simulink model "FOC_fieldWeakening"  (R2023b)
settings: Solver=FixedStepDiscrete  StartTime=0.0  StopTime=3  RelTol=1e-3  EnableMultiTasking=on
InitFcn:
  | mcb_pmsm_fwc_qep_f28379d_data;
model workspace (MAT data in the model file):
  encoderResolution = 2000
  hallOffset = '0.5'
  indexOffset = 850
  polePairs = '4'
values from neighbouring files (symbols this model uses):
  A = 42    [TestigAdder.m]
  dataType = 'single'    [FOC_Param.m]    (also in FOC_simulationParameters.m; mcb_pmsm_fwc_qep_f28379d_data.m; open_loop_control_script.m = fixdt(1,32,17))
  inverter = mcb_updateInverterParameters(pmsm,inverter,target)    [FOC_Param.m]    (also in FOC_simulationParameters.m = mcb_SetInverterParameters('BoostXL-DRV8301'); mcb_pmsm_fwc_qep_f28379d_data.m = mcb_SetInverterParameters('BoostXL-DRV8305'))
  maxMotorCurrent = pmsm.I_rated    [mcb_pmsm_fwc_qep_f28379d_data.m]
  PI_params = mcb_SetControllerParameters(pmsm,inverter,PU_System,T_pwm,Ts,Ts_speed)    [FOC_Param.m]    (also in FOC_simulationParameters.m = mcb_SetControllerParameters(pmsm,inverter,PU_System,T_pwm,2*; mcb_pmsm_fwc_qep_f28379d_data.m = mcb_SetControllerParameters(pmsm,inverter,PU_System,T_pwm,Ts)
  pmsm = mcb_SetPMSMMotorParameters('Teknic2310P')    [FOC_Param.m]    (also in FOC_simulationParameters.m; mcb_pmsm_fwc_qep_f28379d_data.m)
  PU_System = mcb_SetPUSystem(pmsm,inverter)    [FOC_Param.m]    (also in FOC_simulationParameters.m; mcb_pmsm_fwc_qep_f28379d_data.m)
  target = mcb_SetProcessorDetails('F28379D',PWM_frequency)    [FOC_Param.m]    (also in FOC_simulationParameters.m; mcb_pmsm_fwc_qep_f28379d_data.m)
  Ts = T_pwm    (= 5e-05)    [FOC_Param.m]    (also in FOC_simulationParameters.m; mcb_pmsm_fwc_qep_f28379d_data.m; open_loop_control_script.m = T_pwm)
  Ts_speed = 10*Ts    (= 0.0005)    [FOC_Param.m]    (also in FOC_simulationParameters.m = 0.001; mcb_pmsm_fwc_qep_f28379d_data.m = 0.0015)
undefined symbols (not defined in the file or in its folder): Down, GPTRIP1SEL, GPTRIP2SEL, TZ1, TZ2, Up
libraries: simulink x17, mcbcontrolslib x11, c280xlib x10, c2802xlib x7, svdutilitieslib x7, slpidlib x4, c2837xDlib x3, mcbpositiondecoderlib x3, mcbpmsmnonlinearlib x2, svdschedulerlib x2
(part 2 of 3)

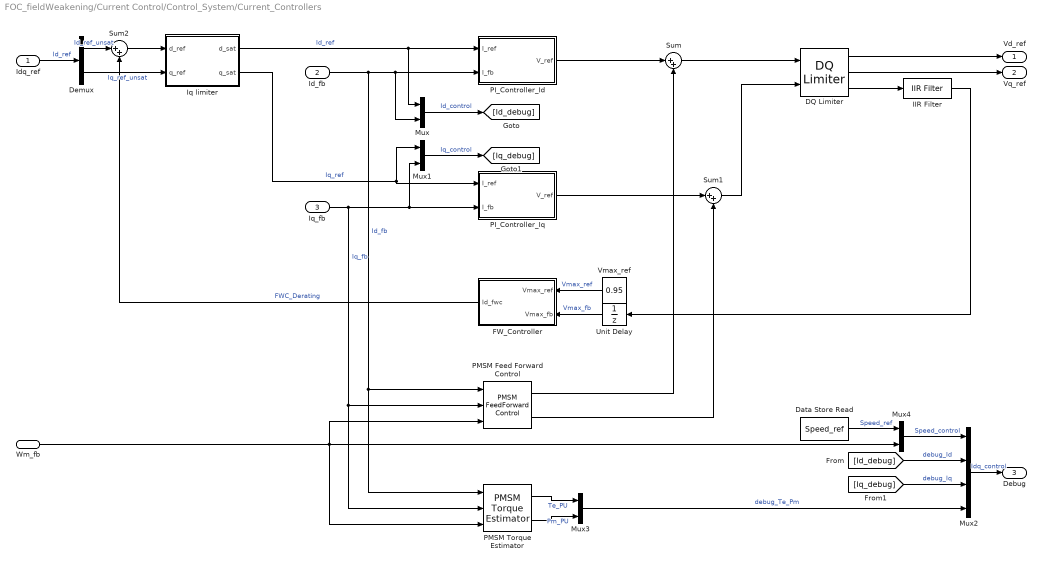
== system FOC_fieldWeakening/Current Control/Control_System/Current_Controllers ==
  Idq_ref : Inport
  Id_fb : Inport  Port=2
  Iq_fb : Inport  Port=3
  Wm_fb : Inport  Port=4
  DQ Limiter : mcbcontrolslib/DQ Limiter  satMethodInputType=Specify via dialog  satMethodSelected=D-Q equivalence  satLimitInputType=Specify via dialog  Vmax=0.95
  Data Store Read : DataStoreRead  DataStoreName=Speed_ref  IndexOptions=Index vector (dialog)  Indices=1  OutputSizes=1
  Demux : Demux  Outputs=2
  FW_Controller : Subsystem
  IIR Filter : mcbcontrolslib/IIR Filter  VariantControl=Low Pass Filter  VariantSelect=Low-pass  Filter_constant=0.01  advancedSettings=off  Ts=50e-6  cutOff_freq=32.1525
  Iq limiter : Subsystem
  Mux{,1,3..4} (4 alike) : Mux  Inputs=2
  Mux2 : Mux
  PI_Controller_Id : Subsystem
  PI_Controller_Iq : Subsystem
  PMSM Feed Forward Control : mcbpmsmnonlinearlib/PMSM FeedForward Control  polePairs=pmsm.p  nonLinearityChoice=Linear model with lumped parameters  Ld=pmsm.Ld  Lq=pmsm.Lq  FluxPM=pmsm.FluxPM  idVec=[-40, -20, 0, 20]  iqVec=[-40, -20, 0, 20, 40]  LdTable=0.2e-3 * ones(4, 5)  LqTable=0.2e-3 * ones(4, 5)  FluxPMTable=6.4e-3 * ones(4, 5)  FluxDTable=[-1.6,-1.6,-1.6,-1.6,-1.6;2.4,2.4,2.4,2.4,2.4;6.4,6.4,6.4,6.4,6.4;10.4,10.4,10.4,10.4,10.4]*1e-3  FluxQTable=[-8,-4,0,4,8;-8,-4,0,4,8;-8,-4,0,4,8;-8,-4,0,4,8]*1e-3  Vsat_input_select=Specify via dialog  v_sat=0.05*PU_System.V_base  Units=Per-Unit (PU)  V_base=PU_System.V_base  I_base=PU_System.I_base  N_base=PU_System.N_base  scaledTables=on
  PMSM Torque Estimator : mcbpmsmnonlinearlib/PMSM Torque Estimator  polePairs=pmsm.p  nonLinearityChoice=Linear model with lumped parameters  Ld=pmsm.Ld  Lq=pmsm.Lq  FluxPM=pmsm.FluxPM  idVec=[-40, -20, 0, 20]  iqVec=[-40, -20, 0, 20, 40]  LdTable=0.2e-3 * ones(4, 5)  LqTable=0.2e-3 * ones(4, 5)  FluxPMTable=6.4e-3 * ones(4, 5)  FluxDTable=[-1.6,-1.6,-1.6,-1.6,-1.6;2.4,2.4,2.4,2.4,2.4;6.4,6.4,6.4,6.4,6.4;10.4,10.4,10.4,10.4,10.4]*1e-3  FluxQTable=[-8,-4,0,4,8;-8,-4,0,4,8;-8,-4,0,4,8;-8,-4,0,4,8]*1e-3  Units=Per-Unit (PU)  V_base=PU_System.V_base  I_base=PU_System.I_base  N_base=PU_System.N_base  T_base=0.82227  P_base=445.3845  scaledTables=on
  Sum : Sum  Inputs=|++
  Sum1 : Sum  Inputs=|++
  Sum2 : Sum  Inputs=|++
  Unit Delay : UnitDelay  SampleTime=-1  HasFrameUpgradeWarning=on
  Vmax_ref : Constant  Value=0.95  OutDataTypeStr=dataType  SampleTime=-1
  Vd_ref : Outport  VectorParamsAs1DForOutWhenUnconnected=off
  Vq_ref : Outport  Port=2  VectorParamsAs1DForOutWhenUnconnected=off
  Debug : Outport  Port=3  VectorParamsAs1DForOutWhenUnconnected=off
  wires:
  Mux/1 -> [Id_debug]  "Id_control"
  Id_fb/1 -> PMSM Torque Estimator/1, PMSM Feed Forward Control/1, Mux/2, PI_Controller_Id/2(I_fb)  "Id_fb"
  Mux1/1 -> [Iq_debug]  "Iq_control"
  DQ Limiter/1 -> Vd_ref/1
  DQ Limiter/2 -> Vq_ref/1
  PI_Controller_Id/1(V_ref) -> Sum/1
  PMSM Torque Estimator/1 -> Mux3/1  "Te_PU"
  FW_Controller/1(Id_fwc) -> Sum2/2  "FWC_Derating"
  Vmax_ref/1 -> FW_Controller/1(Vmax_ref)  "Vmax_ref"
  Iq_fb/1 -> PMSM Torque Estimator/2, PMSM Feed Forward Control/2, PI_Controller_Iq/2(I_fb), Mux1/2  "Iq_fb"
  PI_Controller_Iq/1(V_ref) -> Sum1/1
  Sum1/1 -> DQ Limiter/2
  Sum/1 -> DQ Limiter/1
  Iq limiter/2(q_sat) -> PI_Controller_Iq/1(I_ref), Mux1/1  "Iq_ref"
  Unit Delay/1 -> FW_Controller/2(Vmax_fb)  "Vmax_fb"
  IIR Filter/1 -> Unit Delay/1
  DQ Limiter/3 -> IIR Filter/1
  PMSM Feed Forward Control/1 -> Sum/2
  PMSM Feed Forward Control/2 -> Sum1/2
  Idq_ref/1 -> Demux/1  "Id_ref"
  Mux2/1 -> Debug/1  "Idq_control"
  [Id_debug] -> Mux2/2  "debug_Id"
  [Iq_debug] -> Mux2/3  "debug_Iq"
  PMSM Torque Estimator/2 -> Mux3/2  "Pm_PU"
  Mux3/1 -> Mux2/4  "debug_Te_Pm"
  Mux4/1 -> Mux2/1  "Speed_control"
  Wm_fb/1 -> PMSM Torque Estimator/3, PMSM Feed Forward Control/3, Mux4/2
  Data Store Read/1 -> Mux4/1  "Speed_ref"
  Iq limiter/1(d_sat) -> PI_Controller_Id/1(I_ref), Mux/1  "Id_ref"
  Sum2/1 -> Iq limiter/1(d_ref)
  Demux/1 -> Sum2/1  "Id_ref_unsat"
  Demux/2 -> Iq limiter/2(q_ref)  "Iq_ref_unsat"

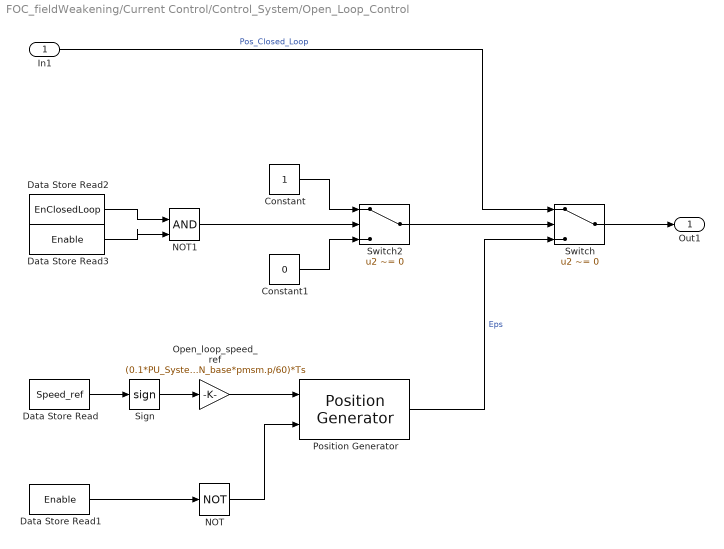
== system FOC_fieldWeakening/Current Control/Control_System/Open_Loop_Control ==
  In1 : Inport
  Constant : Constant  OutDataTypeStr=uint16
  Constant1 : Constant  Value=0  OutDataTypeStr=uint16
  Data Store Read : DataStoreRead  DataStoreName=Speed_ref  IndexOptions=Index vector (dialog)  Indices=1  OutputSizes=1
  Data Store Read1 : DataStoreRead  DataStoreName=Enable  IndexOptions=Index vector (dialog)  Indices=1  OutputSizes=1
  Data Store Read2 : DataStoreRead  DataStoreName=EnClosedLoop  IndexOptions=Index vector (dialog)  Indices=1  OutputSizes=1
  Data Store Read3 : DataStoreRead  DataStoreName=Enable  IndexOptions=Index vector (dialog)  Indices=1  OutputSizes=1
  NOT : Logic  Operator=NOT  IconShape=distinctive  AllPortsSameDT=off  OutDataTypeStr=boolean
  NOT1 : Logic  IconShape=distinctive  AllPortsSameDT=off  OutDataTypeStr=boolean
  Open_loop_speed_ref : Gain  Gain=(0.1*PU_System.N_base*pmsm.p/60)*Ts  ParamDataTypeStr=dataType  OutDataTypeStr=dataType  RndMeth=Simplest
  Position Generator : mcbcontrolslib/Position Generator  AngleOutput=Per-unit  ExternalReset=active high resets to zero  Offset=0
  Sign : Signum
  Switch : Switch  Criteria=u2 ~= 0  Threshold=0.1  SaturateOnIntegerOverflow=off  InputSameDT=off
  Switch2 : Switch  Criteria=u2 ~= 0  SaturateOnIntegerOverflow=off  InputSameDT=off
  Out1 : Outport
  wires:
  Constant1/1 -> Switch2/3
  Constant/1 -> Switch2/1
  In1/1 -> Switch/1  "Pos_Closed_Loop"
  Switch/1 -> Out1/1
  Open_loop_speed_ref/1 -> Position Generator/1
  Switch2/1 -> Switch/2
  Data Store Read/1 -> Sign/1
  Position Generator/1 -> Switch/3  "Eps"
  Data Store Read1/1 -> NOT/1
  NOT/1 -> Position Generator/2
  Data Store Read2/1 -> NOT1/1
  Data Store Read3/1 -> NOT1/2
  NOT1/1 -> Switch2/2
  Sign/1 -> Open_loop_speed_ref/1

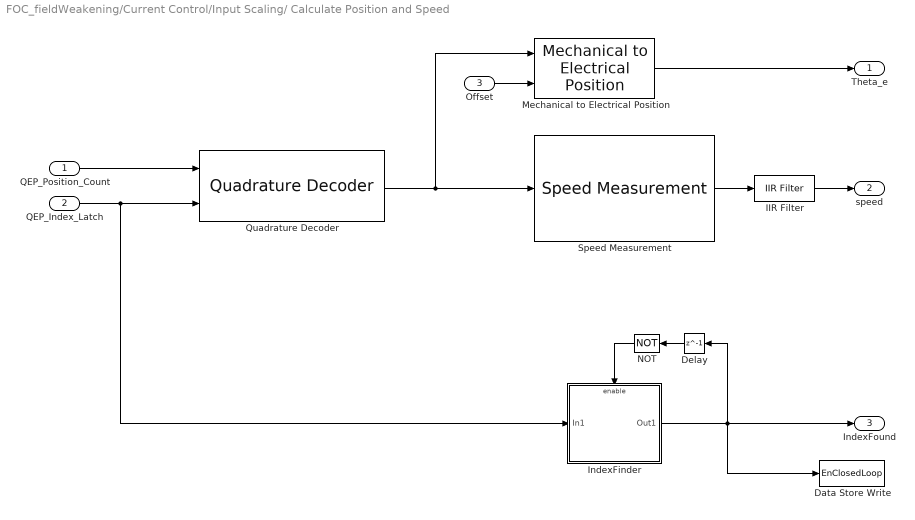
== system FOC_fieldWeakening/Current Control/Input Scaling/ Calculate Position and Speed ==
  QEP_Position_Count : Inport
  QEP_Index_Latch : Inport  Port=2
  Offset : Inport  Port=3
  Data Store Write : DataStoreWrite  DataStoreName=EnClosedLoop  IndexOptions=Index vector (dialog)  Indices=1  OutputSizes=1
  Delay : Delay  DelayLength=1
  IIR Filter : mcbcontrolslib/IIR Filter  VariantControl=Low Pass Filter  VariantSelect=Low-pass  Filter_constant=IIR_filter_speed.coeff_Ts  advancedSettings=off  Ts=50e-6  cutOff_freq=1
  IndexFinder : Subsystem
  Mechanical to Electrical Position : mcbpositiondecoderlib/Mechanical to Electrical Position  PolePairsInputType=Specify via dialog  NrPP=pmsm.p  selectedRange=Per unit  MechOfstInputType=Input port  mechOffsetIn=0  maxAngleIn=1  InputDataType=dataType  VariantSelect=floating-point
  NOT : Logic  Operator=NOT  AllPortsSameDT=off  OutDataTypeStr=boolean
  Quadrature Decoder : mcbpositiondecoderlib/Quadrature Decoder  EncoderSlitsPerRevolution=pmsm.QEPSlits  EncoderCountsPerSlit=4  CounterSize=16 bits  ExternalIndexCount=on  PositionUnit=Per unit  PositionDataType=dataType  ParameterInputType=off  CountsPerRevInverseDataType=single
  Speed Measurement : mcbpositiondecoderlib/Speed Measurement  PositionUnit=Per unit  PositionScalingDatatype=uint32  SpeedCalculationMode=Time interval for speed calculation  SampleTimeAsync=Ts  MaximumApplicationSpeed=6000  SpeedResolution=5e-6  DelayLength=20  MaximumMeasurableSpeed=29999  MeasurableSpeedResolution=1.397e-05  SpeedUnit=Per unit based on dialog  PerUnitSpeed=PU_System.N_base  SpeedDataType=dataType
  Theta_e : Outport  VectorParamsAs1DForOutWhenUnconnected=off
  speed : Outport  Port=2  VectorParamsAs1DForOutWhenUnconnected=off
  IndexFound : Outport  Port=3  InitialOutput=0  VectorParamsAs1DForOutWhenUnconnected=off
  wires:
  Speed Measurement/1 -> IIR Filter/1
  Mechanical to Electrical Position/1 -> Theta_e/1
  QEP_Position_Count/1 -> Quadrature Decoder/1
  Quadrature Decoder/1 -> Mechanical to Electrical Position/1, Speed Measurement/1
  Offset/1 -> Mechanical to Electrical Position/2
  IIR Filter/1 -> speed/1
  Delay/1 -> NOT/1
  NOT/1 -> IndexFinder/Enable
  QEP_Index_Latch/1 -> IndexFinder/1(In1), Quadrature Decoder/2
  IndexFinder/1(Out1) -> Data Store Write/1, Delay/1, IndexFound/1

== system FOC_fieldWeakening/Current Control/Input Scaling/Calculate Phase Currents ==
  Ia_ADC : Inport
  Ib_ADC : Inport  Port=2
  Add : Sum  Inputs=-+
  Data Store Read1 : DataStoreRead  DataStoreName=IaOffset  IndexOptions=Index vector (dialog)  Indices=1  OutputSizes=1
  Data Store Read2 : DataStoreRead  DataStoreName=IbOffset  IndexOptions=Index vector (dialog)  Indices=1  OutputSizes=1
  Data Type Conversion : DataTypeConversion  OutDataTypeStr=int32  ConvertRealWorld=Stored Integer (SI)  RndMeth=Simplest  SaturateOnIntegerOverflow=off
  Data_Type : Subsystem  Variant=on
  Inverting / Non-inverting Current measurement amplifieer : Gain  Gain=inverter.invertingAmp  RndMeth=Simplest  OutDataTypeStr=Inherit: Same as input
  Mux : Mux  Inputs=2
  Mux1 : Mux  Inputs=2
  Iab_meas_PU : Outport  VectorParamsAs1DForOutWhenUnconnected=off
  wires:
  Data Type Conversion/1 -> Add/2
  Add/1 -> Data_Type/1(In1)
  Ia_ADC/1 -> Mux/1
  Ib_ADC/1 -> Mux/2
  Mux/1 -> Data Type Conversion/1
  Mux1/1 -> Add/1
  Data Store Read1/1 -> Mux1/1
  Data Store Read2/1 -> Mux1/2
  Data_Type/1(Out1) -> Inverting / Non-inverting Current measurement amplifieer/1
  Inverting / Non-inverting Current measurement amplifieer/1 -> Iab_meas_PU/1

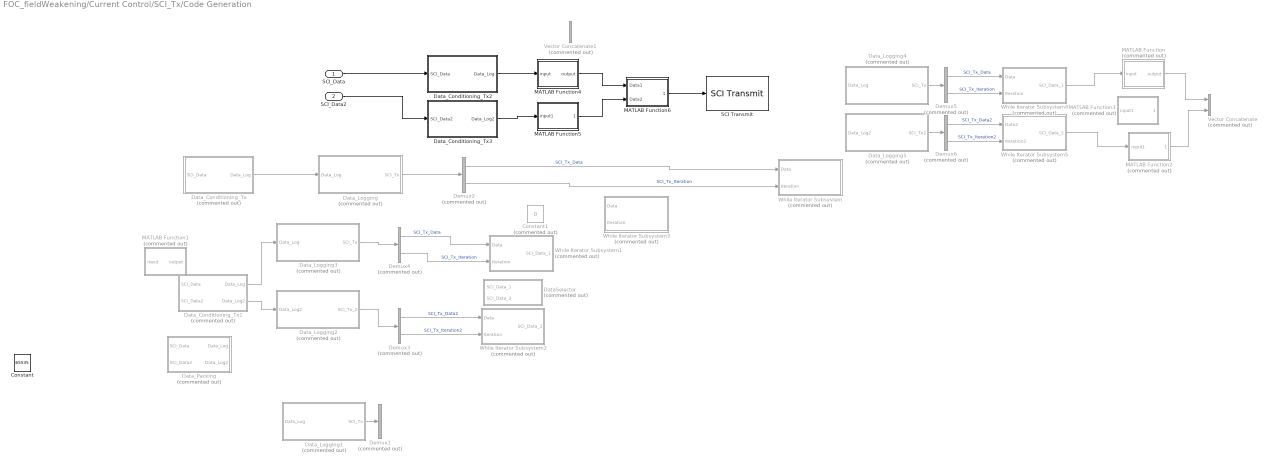
== system FOC_fieldWeakening/Current Control/SCI_Tx/Code Generation ==
  SCI_Data : Inport
  SCI_Data2 : Inport  Port=2
  Constant : Constant  Value=65535  OutDataTypeStr=single
  Constant1 : Constant  Commented=on  Value=0  OutDataTypeStr=uint32
  DataSelector : Subsystem  Commented=on
  Data_Conditioning_Tx : Subsystem  Commented=on  Variant=on
  Data_Conditioning_Tx1 : Subsystem  Commented=on  Variant=on
  Data_Conditioning_Tx2 : Subsystem  Variant=on
  Data_Conditioning_Tx3 : Subsystem  Variant=on
  Data_Logging : Subsystem  Commented=on
  Data_Logging1 : Subsystem  Commented=on
  Data_Logging2 : Subsystem  Commented=on
  Data_Logging3 : Subsystem  Commented=on
  Data_Logging4 : Subsystem  Commented=on
  Data_Logging5 : Subsystem  Commented=on
  Data_Packing : Subsystem  Commented=on  VariantControl=isequal(dataType, 'single')
  Demux{1..6} (6 alike) : Demux  Commented=on  Outputs=2
  MATLAB Function : MATLAB Function  Commented=on  TreatAsAtomicUnit=on
  MATLAB Function1 : MATLAB Function  Commented=on  TreatAsAtomicUnit=on
  MATLAB Function2 : MATLAB Function  Commented=on  TreatAsAtomicUnit=on
  MATLAB Function3 : MATLAB Function  Commented=on  TreatAsAtomicUnit=on
  MATLAB Function4 : MATLAB Function  TreatAsAtomicUnit=on
  MATLAB Function5 : MATLAB Function  TreatAsAtomicUnit=on
  MATLAB Function6 : MATLAB Function  TreatAsAtomicUnit=on
  SCI Transmit : c280xlib/SCI Transmit  sciModule=A  dataHead=''  dataTail=''  frameSize=1  blockingMode=on  outputStatus=off
  Vector Concatenate : Concatenate  Commented=on
  Vector Concatenate1 : Concatenate  Commented=on
  While Iterator Subsystem : Subsystem  Commented=on  TreatAsAtomicUnit=on
  While Iterator Subsystem1 : Subsystem  Commented=on  TreatAsAtomicUnit=on
  While Iterator Subsystem2 : Subsystem  Commented=on  TreatAsAtomicUnit=on
  While Iterator Subsystem3 : Subsystem  Commented=on  TreatAsAtomicUnit=on
  While Iterator Subsystem4 : Subsystem  Commented=on  TreatAsAtomicUnit=on
  While Iterator Subsystem5 : Subsystem  Commented=on  TreatAsAtomicUnit=on
  wires:
  Demux2/2 -> While Iterator Subsystem/2(Iteration)  "SCI_Tx_Iteration"
  Demux2/1 -> While Iterator Subsystem/1(Data)  "SCI_Tx_Data"
  Data_Logging/1(SCI_Tx) -> Demux2/1
  Data_Logging1/1(SCI_Tx) -> Demux1/1
  Data_Logging2/1(SCI_Tx_2) -> Demux3/1
  Demux3/1 -> While Iterator Subsystem2/1(Data)  "SCI_Tx_Data2"
  Demux3/2 -> While Iterator Subsystem2/2(Iteration)  "SCI_Tx_Iteration2"
  Data_Logging3/1(SCI_Tx) -> Demux4/1
  Data_Conditioning_Tx1/1(Data_Log) -> Data_Logging3/1(Data_Log)
  Data_Conditioning_Tx1/2(Data_Log2) -> Data_Logging2/1(Data_Log2)
  Demux4/1 -> While Iterator Subsystem1/1(Data)  "SCI_Tx_Data"
  Demux4/2 -> While Iterator Subsystem1/2(Iteration)  "SCI_Tx_Iteration"
  Data_Conditioning_Tx/1(Data_Log) -> Data_Logging/1(Data_Log)
  SCI_Data/1 -> Data_Conditioning_Tx2/1(SCI_Data)
  Data_Logging4/1(SCI_Tx) -> Demux5/1
  Demux5/1 -> While Iterator Subsystem4/1(Data)  "SCI_Tx_Data"
  Demux5/2 -> While Iterator Subsystem4/2(Iteration)  "SCI_Tx_Iteration"
  Demux6/1 -> While Iterator Subsystem5/1(Data2)  "SCI_Tx_Data2"
  Demux6/2 -> While Iterator Subsystem5/2(Iteration2)  "SCI_Tx_Iteration2"
  Data_Logging5/1(SCI_Tx2) -> Demux6/1
  SCI_Data2/1 -> Data_Conditioning_Tx3/1(SCI_Data2)
  While Iterator Subsystem4/1(SCI_Data_1) -> MATLAB Function/1(input)
  While Iterator Subsystem5/1(SCI_Data_2) -> MATLAB Function2/1(input1)
  MATLAB Function/1(output) -> Vector Concatenate/1
  MATLAB Function2/1(output2) -> Vector Concatenate/2
  Data_Conditioning_Tx2/1(Data_Log) -> MATLAB Function4/1(input)
  Data_Conditioning_Tx3/1(Data_Log2) -> MATLAB Function5/1(input1)
  MATLAB Function4/1(output) -> MATLAB Function6/1(Data1)
  MATLAB Function5/1(output2) -> MATLAB Function6/2(Data2)
  MATLAB Function6/1(DataOut) -> SCI Transmit/1

== system FOC_fieldWeakening/Current Control/SCI_Tx/Simulation ==
  SCI_Data : Inport
  SCI_Data2 : Inport  Port=2
  Demux : Demux  Outputs=2
  Demux1 : Demux  Outputs=2
  Terminator{1..4} (4 alike) : Terminator
  wires:
  SCI_Data/1 -> Demux/1  "DataUT"
  Demux/1 -> Terminator1/1
  Demux1/1 -> Terminator3/1
  Demux1/2 -> Terminator4/1
  Demux/2 -> Terminator2/1
  SCI_Data2/1 -> Demux1/1

== system FOC_fieldWeakening/Hardware Init/Variant Subsystem/Code Generation ==
  note: for BoostXL-DRV8305 connected to LaunchXL-28379D
  note: System Outputs
  note: Enable ADC offset calibration only when motor is not loaded and not rotating due to external factors
  In1 : Inport
  ADC Calib Enable : Constant  Value=target.ADCCalibEnable
  "Calculate ADC Offset " : Subsystem  Priority=1001  TreatAsAtomicUnit=on
  DRV Enable : Subsystem  Priority=1
  Default ADC Offset : Subsystem  Priority=1001  TreatAsAtomicUnit=on
  NOT : Logic  Operator=NOT  IconShape=distinctive  AllPortsSameDT=off  OutDataTypeStr=boolean
  wires:
  In1/1 -> DRV Enable/1(In)
  ADC Calib Enable/1 -> "Calculate ADC Offset "/Enable, NOT/1
  NOT/1 -> Default ADC Offset/Enable

== system FOC_fieldWeakening/Hardware Init/Variant Subsystem/Simulation ==
  In1 : Inport
  Terminator : Terminator
  wires:
  In1/1 -> Terminator/1

== system FOC_fieldWeakening/Heartbeat LED/Heartbeat LED/Code generation ==
  In1 : Inport
  Digital Output : c2837xDlib/Digital Output  GPIO_Number=GPIO32~GPIO39  GPIO_Bit0=off  GPIO_BIT0_Toggle=on  GPIO_Bit1=off  GPIO_BIT1_Toggle=off  GPIO_Bit2=on  GPIO_BIT2_Toggle=on  GPIO_Bit3=off  GPIO_BIT3_Toggle=off  GPIO_Bit4=off  GPIO_BIT4_Toggle=off  GPIO_Bit5=off  GPIO_BIT5_Toggle=off  GPIO_Bit6=off  GPIO_BIT6_Toggle=off  GPIO_Bit7=off  GPIO_BIT7_Toggle=off
  wires:
  In1/1 -> Digital Output/1

== system FOC_fieldWeakening/Heartbeat LED/Heartbeat LED/Simulation ==
  In1 : Inport
  Simulation_Terminator : Terminator
  wires:
  In1/1 -> Simulation_Terminator/1

== system FOC_fieldWeakening/Serial Receive/Data_Conditioning_Rx/Data_Type_Fixed_Point ==
  In1 : Inport
  Data Type Conversion1 : DataTypeConversion  OutDataTypeStr=dataType  RndMeth=Simplest  SaturateOnIntegerOverflow=off
  Data Type Conversion2 : DataTypeConversion  OutDataTypeStr=fixdt(1,32,28)  ConvertRealWorld=Stored Integer (SI)  RndMeth=Simplest  SaturateOnIntegerOverflow=off
  Data Type Conversion3 : DataTypeConversion  OutDataTypeStr=uint16  RndMeth=Simplest  SaturateOnIntegerOverflow=off
  Demux : Demux  Outputs=2
  Out1 : Outport
  Out2 : Outport  Port=2
  wires:
  In1/1 -> Demux/1
  Data Type Conversion1/1 -> Out1/1
  Data Type Conversion2/1 -> Data Type Conversion1/1
  Demux/1 -> Data Type Conversion2/1
  Demux/2 -> Data Type Conversion3/1
  Data Type Conversion3/1 -> Out2/1

== system FOC_fieldWeakening/Serial Receive/Data_Conditioning_Rx/Data_Type_Float ==
  In1 : Inport
  Data Type Conversion2 : DataTypeConversion  OutDataTypeStr=uint16  RndMeth=Simplest  SaturateOnIntegerOverflow=off
  Demux : Demux  Outputs=2
  Out1 : Outport
  Out2 : Outport  Port=2
  wires:
  In1/1 -> Demux/1
  Demux/1 -> Out1/1
  Data Type Conversion2/1 -> Out2/1
  Demux/2 -> Data Type Conversion2/1

== system FOC_fieldWeakening/Serial Receive/SCI_Rx/Code Generation ==
  Data_Type_Fixed_Point : Subsystem  VariantControl=~isequal(dataType, 'single')
  Data_Type_Float : Subsystem  VariantControl=isequal(dataType, 'single')
  Out1 : Outport

== system FOC_fieldWeakening/Serial Receive/SCI_Rx/Simulation ==
  Data Type Conversion2 : DataTypeConversion  OutDataTypeStr=dataType  RndMeth=Simplest  SaturateOnIntegerOverflow=off
  Data_Conditioning_Tx : Subsystem  Variant=on
  Debug_signals : Constant  OutDataTypeStr=uint16  SampleTime=-1
  Enable : Constant  OutDataTypeStr=uint16  SampleTime=-1
  Enable_fwc : Constant  OutDataTypeStr=uint16  SampleTime=-1
  Parse : Subsystem
  Reversal : Step  Time=2
  Speed_Ref_CCW (rpm) : Constant  Value=-1.4*pmsm.N_base  OutDataTypeStr=double  SampleTime=-1
  Speed_Ref_CW (rpm) : Step  Before=0.5*pmsm.N_base  After=1.4*pmsm.N_base
  Switch : Switch  Criteria=u2 > Threshold  SaturateOnIntegerOverflow=off  InputSameDT=off
  rpm2PU : Gain  Gain=1/pmsm.N_base  RndMeth=Simplest  OutDataTypeStr=Inherit: Same as input
  Out1 : Outport
  wires:
  Data_Conditioning_Tx/1(Data) -> Out1/1
  Switch/1 -> rpm2PU/1
  rpm2PU/1 -> Data Type Conversion2/1
  Enable/1 -> Parse/1(Enable_PWM)
  Enable_fwc/1 -> Parse/2(Enable_FWC)
  Debug_signals/1 -> Parse/3(Debug_signals)
  Parse/1(Data) -> Data_Conditioning_Tx/2(In2)
  Data Type Conversion2/1 -> Data_Conditioning_Tx/1(In1)
  Speed_Ref_CCW (rpm)/1 -> Switch/1
  Reversal/1 -> Switch/2
  Speed_Ref_CW (rpm)/1 -> Switch/3

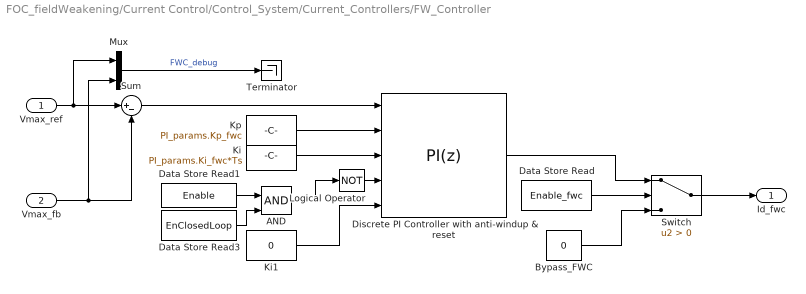
== system FOC_fieldWeakening/Current Control/Control_System/Current_Controllers/FW_Controller ==
  Vmax_ref : Inport
  Vmax_fb : Inport  Port=2
  AND : Logic  IconShape=distinctive  AllPortsSameDT=off  OutDataTypeStr=boolean
  Bypass_FWC : Constant  Value=0  OutDataTypeStr=Inherit: Inherit via back propagation  SampleTime=-1
  Data Store Read : DataStoreRead  DataStoreName=Enable_fwc  IndexOptions=Index vector (dialog)  Indices=1  OutputSizes=1
  Data Store Read1 : DataStoreRead  DataStoreName=Enable  IndexOptions=Index vector (dialog)  Indices=1  OutputSizes=1
  Data Store Read3 : DataStoreRead  DataStoreName=EnClosedLoop  IndexOptions=Index vector (dialog)  Indices=1  OutputSizes=1
  Discrete PI Controller with anti-windup & reset : slpidlib/PID Controller  Controller=PI  Form=Parallel  TimeDomain=Discrete-time  UseExternalTs=off  SampleTime=-1  IntegratorMethod=Forward Euler  FilterMethod=Forward Euler  ControllerParametersSource=external  P=1  I=1  UseKiTs=on  D=0  N=100  UseFilter=on  TunerSelectOption=Transfer Function Based (PID Tuner App)  InitialConditionSource=external  InitialConditionForIntegrator=0  InitialConditionForFilter=0  DifferentiatorICPrevScaledInput=0  ExternalReset=level  TrackingMode=off  Kt=1  LimitOutput=on  SatLimitsSource=internal  UpperSaturationLimit=0  LowerSaturationLimit=-pmsm.I_rated/PU_System.I_base  LinearizeAsGain=on  AntiWindupMode=clamping  Kb=1  LimitIntegrator=off  UpperIntegratorSaturationLimit=inf  LowerIntegratorSaturationLimit=-inf  RndMeth=Simplest  POutMin=[]  POutMax=[]  IOutMin=[]  IOutMax=[]  DOutMin=[]  DOutMax=[]  NOutMin=[]  NOutMax=[]  SumOutMin=[]  SumOutMax=[]  SaturationOutDataTypeStr=Inherit: Inherit via back propagation  SaturationOutMin=[]  SaturationOutMax=[]  PParamMin=[]  PParamMax=[]  IParamMin=[]  IParamMax=[]  DParamMin=[]  DParamMax=[]  NParamMin=[]  NParamMax=[]  KbParamMin=[]  KbParamMax=[]  KtParamMin=[]  KtParamMax=[]  KbOutMin=[]  KbOutMax=[]  KtOutMin=[]  KtOutMax=[]  IntegratorOutMin=[]  IntegratorOutMax=[]  FilterOutMin=[]  FilterOutMax=[]  SumI1OutMin=[]  SumI1OutMax=[]  SumI2OutMin=[]  SumI2OutMax=[]  SumI3OutMin=[]  SumI3OutMax=[]  SumI4OutMin=[]  SumI4OutMax=[]  SumDOutMin=[]  SumDOutMax=[]  DifferentiatorOutMin=[]  DifferentiatorOutMax=[]  FilterDiffOutCoefMin=[]  FilterDiffOutCoefMax=[]  ReciprocalOutMin=[]  ReciprocalOutMax=[]  SumDenOutMin=[]  SumDenOutMax=[]  SumNumOutMin=[]  SumNumOutMax=[]  DivideOutMin=[]  DivideOutMax=[]  UdiffTsProdOutMin=[]  UdiffTsProdOutMax=[]  NTsProdOutMin=[]  NTsProdOutMax=[]  UintegralTsProdOutMin=[]  UintegralTsProdOutMax=[]  UngainTsProdOutMin=[]  UngainTsProdOutMax=[]  ClampingZeroOutDataTypeStr=Inherit: Inherit via back propagation  ClampingZeroOutMin=[]  ClampingZeroOutMax=[]  FilterDenConstantOutDataTypeStr=Inherit: Inherit via back propagation  FilterDenConstantOutMin=[]  FilterDenConstantOutMax=[]  PCopyOutDataTypeStr=Inherit: Inherit via back propagation  PCopyOutMin=[]  PCopyOutMax=[]  NCopyOutDataTypeStr=Inherit: Inherit via back propagation  NCopyOutMin=[]  NCopyOutMax=[]  IntegratorContinuousStateAttributes=''  IntegratorStateMustResolveToSignalObject=off  IntegratorRTWStateStorageClass=Auto  FilterContinuousStateAttributes=''  FilterStateMustResolveToSignalObject=off  FilterRTWStateStorageClass=Auto  ParallelPVariant=ExternalParameters  IdealPVariant=Disabled  IVariant=ExternalParameters  DVariant=Disabled  IntegratorVariant=Discrete  SatVariant=Enabled  AWVariant=DiscClampingParallel  PCopyVariant=Disabled  TRVariant=Disabled  FdbkBlocksVariant=Forward  IdealPFdbkVariant=Disabled  SatFdbkVariant=Disabled  DerivativeFilterVariant=Disabled  NVariant=Disabled  NCopyVariant=Disabled_SignalSpec  FilterICVariant=Disabled  IntegratorICVariant=ExternalICs  ExternalResetVariant=ExternalReset  TRSumVariant=Passthrough  SumFdbkVariant=Disabled  SumVariant=Sum_PI  TsampFilterVariant=InternalTs  TsampNgainVariant=Passthrough  TsampIntegralVariant=Disabled_SignalSpec  ExternalSaturationOutDataTypeStr=Inherit: Same as second input
  Ki : Constant  Value=PI_params.Ki_fwc*Ts  OutDataTypeStr=dataType  SampleTime=-1
  Ki1 : Constant  Value=0  OutDataTypeStr=dataType  SampleTime=-1
  Kp : Constant  Value=PI_params.Kp_fwc  OutDataTypeStr=dataType  SampleTime=-1
  Logical Operator : Logic  Operator=NOT  IconShape=distinctive  AllPortsSameDT=off  OutDataTypeStr=boolean
  Mux : Mux  Inputs=2
  Sum : Sum  Inputs=|+-  OutDataTypeStr=Inherit: Same as first input
  Switch : Switch  Criteria=u2 > Threshold  SaturateOnIntegerOverflow=off  InputSameDT=off
  Terminator : Terminator
  Id_fwc : Outport  VectorParamsAs1DForOutWhenUnconnected=off
  wires:
  Vmax_fb/1 -> Sum/2, Mux/2
  Kp/1 -> Discrete PI Controller with anti-windup & reset/2
  Ki/1 -> Discrete PI Controller with anti-windup & reset/3
  Ki1/1 -> Discrete PI Controller with anti-windup & reset/5
  Mux/1 -> Terminator/1  "FWC_debug"
  Bypass_FWC/1 -> Switch/3
  Switch/1 -> Id_fwc/1
  AND/1 -> Logical Operator/1
  Logical Operator/1 -> Discrete PI Controller with anti-windup & reset/4
  Sum/1 -> Discrete PI Controller with anti-windup & reset/1
  Vmax_ref/1 -> Mux/1, Sum/1
  Data Store Read/1 -> Switch/2
  Discrete PI Controller with anti-windup & reset/1 -> Switch/1
  Data Store Read1/1 -> AND/1
  Data Store Read3/1 -> AND/2

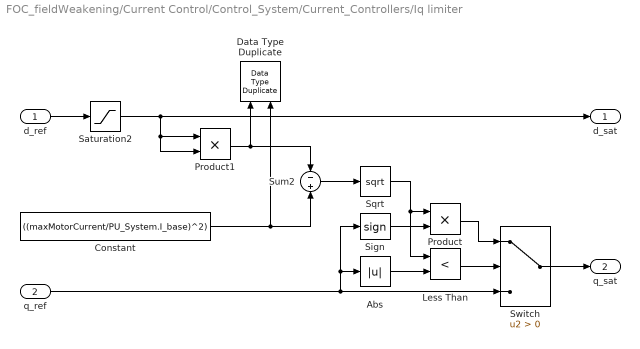
== system FOC_fieldWeakening/Current Control/Control_System/Current_Controllers/Iq limiter ==
  d_ref : Inport
  q_ref : Inport  Port=2
  Abs : Abs  SaturateOnIntegerOverflow=off
  Constant : Constant  Value=((maxMotorCurrent/PU_System.I_base)^2)  OutDataTypeStr=Inherit: Inherit via back propagation  SampleTime=-1
  Data Type Duplicate : DataTypeDuplicate
  Less Than : RelationalOperator  Operator=<  OutDataTypeStr=boolean  RndMeth=Simplest  InputSameDT=off
  Product : Product
  Product1 : Product  RndMeth=Simplest  OutDataTypeStr=Inherit: Same as first input
  Saturation2 : Saturate  UpperLimit=0  LowerLimit=-maxMotorCurrent/PU_System.I_base  RndMeth=Simplest
  Sign : Signum
  Sqrt : Sqrt  RndMeth=Simplest  IntermediateResultsDataTypeStr=Inherit: Inherit from input
  Sum2 : Sum  Inputs=-+  RndMeth=Simplest  OutDataTypeStr=Inherit: Same as first input
  Switch : Switch  Criteria=u2 > Threshold  SaturateOnIntegerOverflow=off  InputSameDT=off
  d_sat : Outport
  q_sat : Outport  Port=2
  wires:
  Product/1 -> Switch/1
  Sign/1 -> Product/2
  d_ref/1 -> Saturation2/1
  Less Than/1 -> Switch/2
  Abs/1 -> Less Than/2
  Sum2/1 -> Sqrt/1
  Switch/1 -> q_sat/1
  Sqrt/1 -> Less Than/1, Product/1
  Constant/1 -> Sum2/2, Data Type Duplicate/2
  Saturation2/1 -> Product1/2, Product1/1, d_sat/1
  q_ref/1 -> Sign/1, Abs/1, Switch/3
  Product1/1 -> Sum2/1, Data Type Duplicate/1

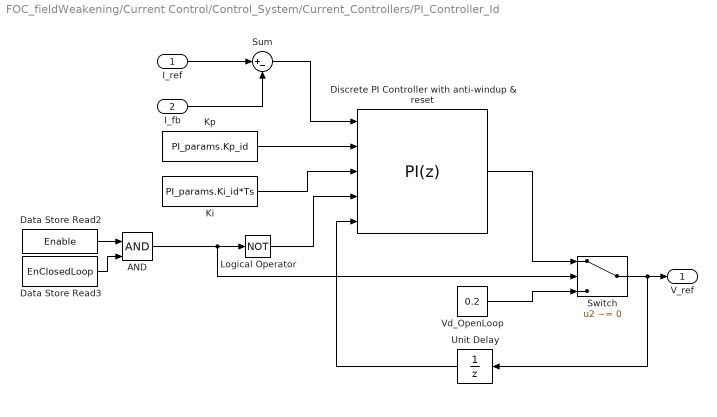
== system FOC_fieldWeakening/Current Control/Control_System/Current_Controllers/PI_Controller_Id ==
  I_ref : Inport
  I_fb : Inport  Port=2
  AND : Logic  IconShape=distinctive  AllPortsSameDT=off  OutDataTypeStr=boolean
  Data Store Read2 : DataStoreRead  DataStoreName=Enable  IndexOptions=Index vector (dialog)  Indices=1  OutputSizes=1
  Data Store Read3 : DataStoreRead  DataStoreName=EnClosedLoop  IndexOptions=Index vector (dialog)  Indices=1  OutputSizes=1
  Discrete PI Controller with anti-windup & reset : slpidlib/PID Controller  Controller=PI  Form=Parallel  TimeDomain=Discrete-time  UseExternalTs=off  SampleTime=-1  IntegratorMethod=Forward Euler  FilterMethod=Forward Euler  ControllerParametersSource=external  P=1  I=1  UseKiTs=on  D=0  N=100  UseFilter=on  TunerSelectOption=Transfer Function Based (PID Tuner App)  InitialConditionSource=external  InitialConditionForIntegrator=0  InitialConditionForFilter=0  DifferentiatorICPrevScaledInput=0  ExternalReset=level  TrackingMode=off  Kt=1  LimitOutput=on  SatLimitsSource=internal  UpperSaturationLimit=1  LowerSaturationLimit=-1  LinearizeAsGain=on  AntiWindupMode=clamping  Kb=1  LimitIntegrator=off  UpperIntegratorSaturationLimit=inf  LowerIntegratorSaturationLimit=-inf  RndMeth=Simplest  POutMin=[]  POutMax=[]  IOutMin=[]  IOutMax=[]  DOutMin=[]  DOutMax=[]  NOutMin=[]  NOutMax=[]  SumOutMin=[]  SumOutMax=[]  SaturationOutDataTypeStr=Inherit: Inherit via back propagation  SaturationOutMin=[]  SaturationOutMax=[]  PParamMin=[]  PParamMax=[]  IParamMin=[]  IParamMax=[]  DParamMin=[]  DParamMax=[]  NParamMin=[]  NParamMax=[]  KbParamMin=[]  KbParamMax=[]  KtParamMin=[]  KtParamMax=[]  KbOutMin=[]  KbOutMax=[]  KtOutMin=[]  KtOutMax=[]  IntegratorOutMin=[]  IntegratorOutMax=[]  FilterOutMin=[]  FilterOutMax=[]  SumI1OutMin=[]  SumI1OutMax=[]  SumI2OutMin=[]  SumI2OutMax=[]  SumI3OutMin=[]  SumI3OutMax=[]  SumI4OutMin=[]  SumI4OutMax=[]  SumDOutMin=[]  SumDOutMax=[]  DifferentiatorOutMin=[]  DifferentiatorOutMax=[]  FilterDiffOutCoefMin=[]  FilterDiffOutCoefMax=[]  ReciprocalOutMin=[]  ReciprocalOutMax=[]  SumDenOutMin=[]  SumDenOutMax=[]  SumNumOutMin=[]  SumNumOutMax=[]  DivideOutMin=[]  DivideOutMax=[]  UdiffTsProdOutMin=[]  UdiffTsProdOutMax=[]  NTsProdOutMin=[]  NTsProdOutMax=[]  UintegralTsProdOutMin=[]  UintegralTsProdOutMax=[]  UngainTsProdOutMin=[]  UngainTsProdOutMax=[]  ClampingZeroOutDataTypeStr=Inherit: Inherit via back propagation  ClampingZeroOutMin=[]  ClampingZeroOutMax=[]  FilterDenConstantOutDataTypeStr=Inherit: Inherit via back propagation  FilterDenConstantOutMin=[]  FilterDenConstantOutMax=[]  PCopyOutDataTypeStr=Inherit: Inherit via back propagation  PCopyOutMin=[]  PCopyOutMax=[]  NCopyOutDataTypeStr=Inherit: Inherit via back propagation  NCopyOutMin=[]  NCopyOutMax=[]  IntegratorContinuousStateAttributes=''  IntegratorStateMustResolveToSignalObject=off  IntegratorRTWStateStorageClass=Auto  FilterContinuousStateAttributes=''  FilterStateMustResolveToSignalObject=off  FilterRTWStateStorageClass=Auto  ParallelPVariant=ExternalParameters  IdealPVariant=Disabled  IVariant=ExternalParameters  DVariant=Disabled  IntegratorVariant=Discrete  SatVariant=Enabled  AWVariant=DiscClampingParallel  PCopyVariant=Disabled  TRVariant=Disabled  FdbkBlocksVariant=Forward  IdealPFdbkVariant=Disabled  SatFdbkVariant=Disabled  DerivativeFilterVariant=Disabled  NVariant=Disabled  NCopyVariant=Disabled_SignalSpec  FilterICVariant=Disabled  IntegratorICVariant=ExternalICs  ExternalResetVariant=ExternalReset  TRSumVariant=Passthrough  SumFdbkVariant=Disabled  SumVariant=Sum_PI  TsampFilterVariant=InternalTs  TsampNgainVariant=Passthrough  TsampIntegralVariant=Disabled_SignalSpec  ExternalSaturationOutDataTypeStr=Inherit: Same as second input
  Ki : Constant  Value=PI_params.Ki_id*Ts  OutDataTypeStr=dataType  SampleTime=-1
  Kp : Constant  Value=PI_params.Kp_id  OutDataTypeStr=dataType  SampleTime=-1
  Logical Operator : Logic  Operator=NOT  IconShape=distinctive  AllPortsSameDT=off  OutDataTypeStr=boolean
  Sum : Sum  Inputs=|+-  OutDataTypeStr=Inherit: Same as first input
  Switch : Switch  Criteria=u2 ~= 0  RndMeth=Simplest  SaturateOnIntegerOverflow=off  InputSameDT=off
  Unit Delay : UnitDelay  SampleTime=-1  HasFrameUpgradeWarning=on
  Vd_OpenLoop : Constant  Value=0.2  OutDataTypeStr=dataType  SampleTime=-1
  V_ref : Outport  VectorParamsAs1DForOutWhenUnconnected=off
  wires:
  I_fb/1 -> Sum/2
  Discrete PI Controller with anti-windup & reset/1 -> Switch/1
  I_ref/1 -> Sum/1
  Vd_OpenLoop/1 -> Switch/3
  Ki/1 -> Discrete PI Controller with anti-windup & reset/3
  Unit Delay/1 -> Discrete PI Controller with anti-windup & reset/5
  Logical Operator/1 -> Discrete PI Controller with anti-windup & reset/4
  Sum/1 -> Discrete PI Controller with anti-windup & reset/1
  Kp/1 -> Discrete PI Controller with anti-windup & reset/2
  Switch/1 -> V_ref/1, Unit Delay/1
  AND/1 -> Logical Operator/1, Switch/2
  Data Store Read2/1 -> AND/1
  Data Store Read3/1 -> AND/2

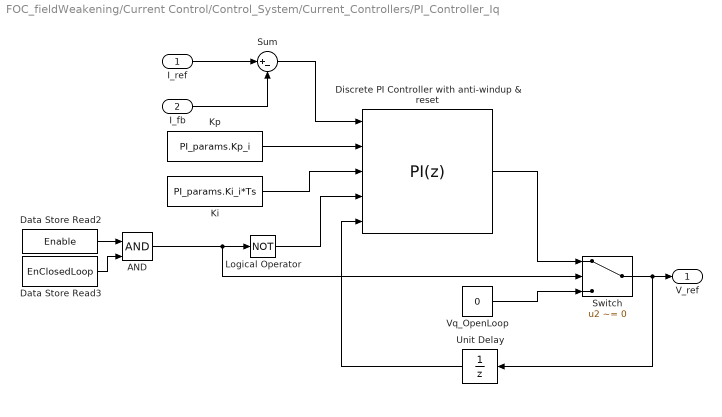
== system FOC_fieldWeakening/Current Control/Control_System/Current_Controllers/PI_Controller_Iq ==
  I_ref : Inport
  I_fb : Inport  Port=2
  AND : Logic  IconShape=distinctive  AllPortsSameDT=off  OutDataTypeStr=boolean
  Data Store Read2 : DataStoreRead  DataStoreName=Enable  IndexOptions=Index vector (dialog)  Indices=1  OutputSizes=1
  Data Store Read3 : DataStoreRead  DataStoreName=EnClosedLoop  IndexOptions=Index vector (dialog)  Indices=1  OutputSizes=1
  Discrete PI Controller with anti-windup & reset : slpidlib/PID Controller  Controller=PI  Form=Parallel  TimeDomain=Discrete-time  UseExternalTs=off  SampleTime=-1  IntegratorMethod=Forward Euler  FilterMethod=Forward Euler  ControllerParametersSource=external  P=1  I=1  UseKiTs=on  D=0  N=100  UseFilter=on  TunerSelectOption=Transfer Function Based (PID Tuner App)  InitialConditionSource=external  InitialConditionForIntegrator=0  InitialConditionForFilter=0  DifferentiatorICPrevScaledInput=0  ExternalReset=level  TrackingMode=off  Kt=1  LimitOutput=on  SatLimitsSource=internal  UpperSaturationLimit=1  LowerSaturationLimit=-1  LinearizeAsGain=on  AntiWindupMode=clamping  Kb=1  LimitIntegrator=off  UpperIntegratorSaturationLimit=inf  LowerIntegratorSaturationLimit=-inf  RndMeth=Simplest  POutMin=[]  POutMax=[]  IOutMin=[]  IOutMax=[]  DOutMin=[]  DOutMax=[]  NOutMin=[]  NOutMax=[]  SumOutMin=[]  SumOutMax=[]  SaturationOutDataTypeStr=Inherit: Inherit via back propagation  SaturationOutMin=[]  SaturationOutMax=[]  PParamMin=[]  PParamMax=[]  IParamMin=[]  IParamMax=[]  DParamMin=[]  DParamMax=[]  NParamMin=[]  NParamMax=[]  KbParamMin=[]  KbParamMax=[]  KtParamMin=[]  KtParamMax=[]  KbOutMin=[]  KbOutMax=[]  KtOutMin=[]  KtOutMax=[]  IntegratorOutMin=[]  IntegratorOutMax=[]  FilterOutMin=[]  FilterOutMax=[]  SumI1OutMin=[]  SumI1OutMax=[]  SumI2OutMin=[]  SumI2OutMax=[]  SumI3OutMin=[]  SumI3OutMax=[]  SumI4OutMin=[]  SumI4OutMax=[]  SumDOutMin=[]  SumDOutMax=[]  DifferentiatorOutMin=[]  DifferentiatorOutMax=[]  FilterDiffOutCoefMin=[]  FilterDiffOutCoefMax=[]  ReciprocalOutMin=[]  ReciprocalOutMax=[]  SumDenOutMin=[]  SumDenOutMax=[]  SumNumOutMin=[]  SumNumOutMax=[]  DivideOutMin=[]  DivideOutMax=[]  UdiffTsProdOutMin=[]  UdiffTsProdOutMax=[]  NTsProdOutMin=[]  NTsProdOutMax=[]  UintegralTsProdOutMin=[]  UintegralTsProdOutMax=[]  UngainTsProdOutMin=[]  UngainTsProdOutMax=[]  ClampingZeroOutDataTypeStr=Inherit: Inherit via back propagation  ClampingZeroOutMin=[]  ClampingZeroOutMax=[]  FilterDenConstantOutDataTypeStr=Inherit: Inherit via back propagation  FilterDenConstantOutMin=[]  FilterDenConstantOutMax=[]  PCopyOutDataTypeStr=Inherit: Inherit via back propagation  PCopyOutMin=[]  PCopyOutMax=[]  NCopyOutDataTypeStr=Inherit: Inherit via back propagation  NCopyOutMin=[]  NCopyOutMax=[]  IntegratorContinuousStateAttributes=''  IntegratorStateMustResolveToSignalObject=off  IntegratorRTWStateStorageClass=Auto  FilterContinuousStateAttributes=''  FilterStateMustResolveToSignalObject=off  FilterRTWStateStorageClass=Auto  ParallelPVariant=ExternalParameters  IdealPVariant=Disabled  IVariant=ExternalParameters  DVariant=Disabled  IntegratorVariant=Discrete  SatVariant=Enabled  AWVariant=DiscClampingParallel  PCopyVariant=Disabled  TRVariant=Disabled  FdbkBlocksVariant=Forward  IdealPFdbkVariant=Disabled  SatFdbkVariant=Disabled  DerivativeFilterVariant=Disabled  NVariant=Disabled  NCopyVariant=Disabled_SignalSpec  FilterICVariant=Disabled  IntegratorICVariant=ExternalICs  ExternalResetVariant=ExternalReset  TRSumVariant=Passthrough  SumFdbkVariant=Disabled  SumVariant=Sum_PI  TsampFilterVariant=InternalTs  TsampNgainVariant=Passthrough  TsampIntegralVariant=Disabled_SignalSpec  ExternalSaturationOutDataTypeStr=Inherit: Same as second input
  Ki : Constant  Value=PI_params.Ki_i*Ts  OutDataTypeStr=dataType  SampleTime=-1
  Kp : Constant  Value=PI_params.Kp_i  OutDataTypeStr=dataType  SampleTime=-1
  Logical Operator : Logic  Operator=NOT  IconShape=distinctive  AllPortsSameDT=off  OutDataTypeStr=boolean
  Sum : Sum  Inputs=|+-  OutDataTypeStr=Inherit: Same as first input
  Switch : Switch  Criteria=u2 ~= 0  RndMeth=Simplest  SaturateOnIntegerOverflow=off  InputSameDT=off
  Unit Delay : UnitDelay  SampleTime=-1  HasFrameUpgradeWarning=on
  Vq_OpenLoop : Constant  Value=0  OutDataTypeStr=dataType  SampleTime=-1
  V_ref : Outport  VectorParamsAs1DForOutWhenUnconnected=off
  wires:
  I_fb/1 -> Sum/2
  Discrete PI Controller with anti-windup & reset/1 -> Switch/1
  I_ref/1 -> Sum/1
  Vq_OpenLoop/1 -> Switch/3
  Ki/1 -> Discrete PI Controller with anti-windup & reset/3
  Unit Delay/1 -> Discrete PI Controller with anti-windup & reset/5
  Logical Operator/1 -> Discrete PI Controller with anti-windup & reset/4
  Sum/1 -> Discrete PI Controller with anti-windup & reset/1
  Kp/1 -> Discrete PI Controller with anti-windup & reset/2
  Switch/1 -> V_ref/1, Unit Delay/1
  AND/1 -> Logical Operator/1, Switch/2
  Data Store Read2/1 -> AND/1
  Data Store Read3/1 -> AND/2

== system FOC_fieldWeakening/Current Control/Input Scaling/ Calculate Position and Speed/IndexFinder ==
  In1 : Inport
  Enable : EnablePort
  AND : Logic  AllPortsSameDT=off  OutDataTypeStr=boolean
  Compare To Constant : simulink/Logic and Bit Operations/Compare To Constant  relop===  const=0  OutDataTypeStr=boolean
  Compare To Constant1 : simulink/Logic and Bit Operations/Compare To Constant  relop=>  const=0  OutDataTypeStr=boolean
  Delay3 : Delay  DelayLength=1
  Out1 : Outport
  wires:
  In1/1 -> Delay3/1, Compare To Constant1/1
  Compare To Constant1/1 -> AND/2
  Compare To Constant/1 -> AND/1
  Delay3/1 -> Compare To Constant/1
  AND/1 -> Out1/1

== system FOC_fieldWeakening/Current Control/Input Scaling/Calculate Phase Currents/Data_Type ==
  In1 : Inport
  Data_Type_Fixed_Point : Subsystem  VariantControl=~isequal(dataType,'single')
  Data_Type_Float : Subsystem  VariantControl=isequal(dataType,'single')
  Out1 : Outport

== system FOC_fieldWeakening/Current Control/SCI_Tx/Code Generation/DataSelector ==
  SCI_Data_1 : Inport
  SCI_Data_2 : Inport  Port=2
  Counter Limited : simulink/Sources/Counter Limited  uplimit=599  tsamp=-1
  If : If  IfExpression=u1 < 300
  SCI Transmit : c280xlib/SCI Transmit  sciModule=A  dataHead=''  dataTail=''  frameSize=1  blockingMode=on  outputStatus=off
  SCI Transmit1 : c280xlib/SCI Transmit  Commented=on  sciModule=A  dataHead=''  dataTail=''  frameSize=1  blockingMode=on  outputStatus=off
  Select1 : Subsystem  TreatAsAtomicUnit=on
  Select2 : Subsystem  TreatAsAtomicUnit=on
  wires:
  Counter Limited/1 -> If/1
  SCI_Data_1/1 -> Select1/1(SCI_Data_1)
  If/1 -> Select1/Action
  If/2 -> Select2/Action
  SCI_Data_2/1 -> Select2/1(SCI_Data_2)
  Select1/1(SCI_Data_Transmit) -> SCI Transmit/1

== system FOC_fieldWeakening/Current Control/SCI_Tx/Code Generation/Data_Conditioning_Tx ==
  SCI_Data : Inport
  Data_Type_Fixed_Point : Subsystem  VariantControl=~isequal(dataType,'single')
  Data_Type_Float : Subsystem  VariantControl=isequal(dataType, 'single')
  Data_Log : Outport

== system FOC_fieldWeakening/Current Control/SCI_Tx/Code Generation/Data_Conditioning_Tx1 ==
  SCI_Data : Inport
  SCI_Data2 : Inport  Port=2
  Data_Type_Fixed_Point : Subsystem  VariantControl=~isequal(dataType,'single')
  Data_Type_Float : Subsystem  VariantControl=isequal(dataType, 'single')
  Data_Log : Outport
  Data_Log2 : Outport  Port=2

== system FOC_fieldWeakening/Current Control/SCI_Tx/Code Generation/Data_Conditioning_Tx2 ==
  SCI_Data : Inport
  Data_Type_Fixed_Point : Subsystem  VariantControl=~isequal(dataType,'single')
  Data_Type_Float : Subsystem  VariantControl=isequal(dataType, 'single')
  Data_Log : Outport

== system FOC_fieldWeakening/Current Control/SCI_Tx/Code Generation/Data_Conditioning_Tx3 ==
  SCI_Data2 : Inport
  Data_Type_Fixed_Point : Subsystem  VariantControl=~isequal(dataType,'single')
  Data_Type_Float : Subsystem  VariantControl=isequal(dataType, 'single')
  Data_Log2 : Outport

== system FOC_fieldWeakening/Current Control/SCI_Tx/Code Generation/Data_Logging ==
  note: Fast Serial Data Monitoring (32-bit)
  Data_Log : Inport
  Counter Limited : simulink/Sources/Counter Limited  uplimit=600-1  tsamp=-1
  Data : Subsystem  TreatAsAtomicUnit=on
  End : Subsystem  TreatAsAtomicUnit=on
  If : If  IfExpression=u1 == 0  ElseIfExpressions=u1 == 599
  Merge : Merge  Inputs=3
  Merge1 : Merge  Inputs=3
  Mux : Mux  Inputs=2
  Start : Subsystem  TreatAsAtomicUnit=on
  Width : Width  OutDataTypeMode=All ports same datatype  DataType=uint16
  SCI_Tx : Outport
  wires:
  If/3 -> Data/Action
  Data/1(Data_out) -> Merge/3
  Width/1 -> Data/2(Data_width), Start/2(Data_width), End/2(Data_width)
  Merge/1 -> Mux/1  "SCI_Tx_Data"
  Counter Limited/1 -> If/1
  Start/2(Iteration) -> Merge1/1
  Start/1(Data_out) -> Merge/1
  If/2 -> End/Action
  Merge1/1 -> Mux/2  "SCI_Tx_Iteration"
  If/1 -> Start/Action
  End/1(Data_out) -> Merge/2
  End/2(Iteration) -> Merge1/2
  Data/2(Iteration) -> Merge1/3
  Mux/1 -> SCI_Tx/1
  Data_Log/1 -> Width/1, Start/1(Data), End/1(Data), Data/1(Data)

== system FOC_fieldWeakening/Current Control/SCI_Tx/Code Generation/Data_Logging1 ==
  note: Fast Serial Data Monitoring (32-bit)
  Data_Log : Inport
  Counter Limited : simulink/Sources/Counter Limited  uplimit=300-1  tsamp=-1
  Data : Subsystem  TreatAsAtomicUnit=on
  End : Subsystem  TreatAsAtomicUnit=on
  If : If  IfExpression=u1 == 0  ElseIfExpressions=u1 == 299
  Merge : Merge  Inputs=3
  Merge1 : Merge  Inputs=3
  Mux : Mux  Inputs=2
  Start : Subsystem  TreatAsAtomicUnit=on
  Width : Width  OutDataTypeMode=All ports same datatype  DataType=uint16
  SCI_Tx : Outport
  wires:
  If/3 -> Data/Action
  Data/1(Data_out) -> Merge/3
  Width/1 -> Data/2(Data_width), Start/2(Data_width), End/2(Data_width)
  Merge/1 -> Mux/1  "SCI_Tx_Data"
  Counter Limited/1 -> If/1
  Start/2(Iteration) -> Merge1/1
  Start/1(Data_out) -> Merge/1
  If/2 -> End/Action
  Merge1/1 -> Mux/2  "SCI_Tx_Iteration"
  If/1 -> Start/Action
  End/1(Data_out) -> Merge/2
  End/2(Iteration) -> Merge1/2
  Data/2(Iteration) -> Merge1/3
  Mux/1 -> SCI_Tx/1
  Data_Log/1 -> Width/1, Start/1(Data), End/1(Data), Data/1(Data)

== system FOC_fieldWeakening/Current Control/SCI_Tx/Code Generation/Data_Logging2 ==
  note: Fast Serial Data Monitoring (32-bit)
  Data_Log2 : Inport
  Counter Limited : simulink/Sources/Counter Limited  uplimit=300-1  tsamp=-1
  Data : Subsystem  TreatAsAtomicUnit=on
  End : Subsystem  TreatAsAtomicUnit=on
  If : If  IfExpression=u1 == 0  ElseIfExpressions=u1 == 299
  Merge : Merge  Inputs=3
  Merge1 : Merge  Inputs=3
  Mux : Mux  Inputs=2
  Start : Subsystem  TreatAsAtomicUnit=on
  Width : Width  OutDataTypeMode=All ports same datatype  DataType=uint16
  SCI_Tx_2 : Outport
  wires:
  If/3 -> Data/Action
  Data/1(Data_out) -> Merge/3
  Width/1 -> Data/2(Data_width), Start/2(Data_width), End/2(Data_width)
  Merge/1 -> Mux/1  "SCI_Tx_Data2"
  Counter Limited/1 -> If/1
  Start/2(Iteration) -> Merge1/1
  Start/1(Data_out) -> Merge/1
  If/2 -> End/Action
  Merge1/1 -> Mux/2  "SCI_Tx_Iteration2"
  If/1 -> Start/Action
  End/1(Data_out) -> Merge/2
  End/2(Iteration) -> Merge1/2
  Data/2(Iteration) -> Merge1/3
  Mux/1 -> SCI_Tx_2/1
  Data_Log2/1 -> Width/1, Start/1(Data), End/1(Data), Data/1(Data)

== system FOC_fieldWeakening/Current Control/SCI_Tx/Code Generation/Data_Logging3 ==
  note: Fast Serial Data Monitoring (32-bit)
  Data_Log : Inport
  Counter Limited : simulink/Sources/Counter Limited  uplimit=300-1  tsamp=-1
  Data : Subsystem  TreatAsAtomicUnit=on
  End : Subsystem  TreatAsAtomicUnit=on
  If : If  IfExpression=u1 == 0  ElseIfExpressions=u1 == 299
  Merge : Merge  Inputs=3
  Merge1 : Merge  Inputs=3
  Mux : Mux  Inputs=2
  Start : Subsystem  TreatAsAtomicUnit=on
  Width : Width  OutDataTypeMode=All ports same datatype  DataType=uint16
  SCI_Tx : Outport
  wires:
  If/3 -> Data/Action
  Data/1(Data_out) -> Merge/3
  Width/1 -> Data/2(Data_width), Start/2(Data_width), End/2(Data_width)
  Merge/1 -> Mux/1  "SCI_Tx_Data"
  Counter Limited/1 -> If/1
  Start/2(Iteration) -> Merge1/1
  Start/1(Data_out) -> Merge/1
  If/2 -> End/Action
  Merge1/1 -> Mux/2  "SCI_Tx_Iteration"
  If/1 -> Start/Action
  End/1(Data_out) -> Merge/2
  End/2(Iteration) -> Merge1/2
  Data/2(Iteration) -> Merge1/3
  Mux/1 -> SCI_Tx/1
  Data_Log/1 -> Width/1, Start/1(Data), End/1(Data), Data/1(Data)

== system FOC_fieldWeakening/Current Control/SCI_Tx/Code Generation/Data_Logging4 ==
  note: Fast Serial Data Monitoring (32-bit)
  Data_Log : Inport
  Counter Limited : simulink/Sources/Counter Limited  uplimit=600-1  tsamp=-1
  Data : Subsystem  TreatAsAtomicUnit=on
  End : Subsystem  TreatAsAtomicUnit=on
  If : If  IfExpression=u1 == 0  ElseIfExpressions=u1 == 599
  Merge : Merge  Inputs=3
  Merge1 : Merge  Inputs=3
  Mux : Mux  Inputs=2
  Start : Subsystem  TreatAsAtomicUnit=on
  Width : Width  OutDataTypeMode=All ports same datatype  DataType=uint16
  SCI_Tx : Outport
  wires:
  If/3 -> Data/Action
  Data/1(Data_out) -> Merge/3
  Width/1 -> Data/2(Data_width), Start/2(Data_width), End/2(Data_width)
  Merge/1 -> Mux/1  "SCI_Tx_Data"
  Counter Limited/1 -> If/1
  Start/2(Iteration) -> Merge1/1
  Start/1(Data_out) -> Merge/1
  If/2 -> End/Action
  Merge1/1 -> Mux/2  "SCI_Tx_Iteration"
  If/1 -> Start/Action
  End/1(Data_out) -> Merge/2
  End/2(Iteration) -> Merge1/2
  Data/2(Iteration) -> Merge1/3
  Mux/1 -> SCI_Tx/1
  Data_Log/1 -> Width/1, Start/1(Data), End/1(Data), Data/1(Data)

== system FOC_fieldWeakening/Current Control/SCI_Tx/Code Generation/Data_Logging5 ==
  note: Fast Serial Data Monitoring (32-bit)
  Data_Log2 : Inport
  Counter Limited : simulink/Sources/Counter Limited  uplimit=600-1  tsamp=-1
  Data : Subsystem  TreatAsAtomicUnit=on
  End : Subsystem  TreatAsAtomicUnit=on
  If : If  IfExpression=u1 == 0  ElseIfExpressions=u1 == 599
  Merge : Merge  Inputs=3
  Merge1 : Merge  Inputs=3
  Mux : Mux  Inputs=2
  Start : Subsystem  TreatAsAtomicUnit=on
  Width : Width  OutDataTypeMode=All ports same datatype  DataType=uint16
  SCI_Tx2 : Outport
  wires:
  If/3 -> Data/Action
  Data/1(Data_out) -> Merge/3
  Width/1 -> Data/2(Data_width), Start/2(Data_width), End/2(Data_width)
  Merge/1 -> Mux/1  "SCI_Tx_Data"
  Counter Limited/1 -> If/1
  Start/2(Iteration) -> Merge1/1
  Start/1(Data_out) -> Merge/1
  If/2 -> End/Action
  Merge1/1 -> Mux/2  "SCI_Tx_Iteration"
  If/1 -> Start/Action
  End/1(Data_out) -> Merge/2
  End/2(Iteration) -> Merge1/2
  Data/2(Iteration) -> Merge1/3
  Mux/1 -> SCI_Tx2/1
  Data_Log2/1 -> Width/1, Start/1(Data), End/1(Data), Data/1(Data)

== system FOC_fieldWeakening/Current Control/SCI_Tx/Code Generation/Data_Packing ==
  SCI_Data : Inport
  SCI_Data2 : Inport  Port=2
  Byte Pack : svdutilitieslib/Byte Pack  maskPackedDataType=uint32  datatypes={'single'}  byteAlign=4  blockPlatform=tic2000
  Byte Pack1 : svdutilitieslib/Byte Pack  maskPackedDataType=uint32  datatypes={'single'}  byteAlign=4  blockPlatform=tic2000
  Data_Log : Outport
  Data_Log2 : Outport  Port=2
  wires:
  Byte Pack/1 -> Data_Log/1
  SCI_Data/1 -> Byte Pack/1
  SCI_Data2/1 -> Byte Pack1/1
  Byte Pack1/1 -> Data_Log2/1

== system FOC_fieldWeakening/Current Control/SCI_Tx/Code Generation/While Iterator Subsystem ==
  Data : Inport
  Iteration : Inport  Port=2
  Add : Sum  Inputs=+-  OutDataTypeStr=Inherit: Same as first input
  Index Vector : MultiPortSwitch  Inputs=1  SaturateOnIntegerOverflow=off  InputSameDT=off
  SCI Transmit : c280xlib/SCI Transmit  sciModule=A  dataHead=''  dataTail=''  frameSize=1  blockingMode=on  outputStatus=off
  While Iterator : WhileIterator  MaxIters=-1  WhileBlockType=do-while  ShowIterationPort=on  OutputDataType=int16
  wires:
  While Iterator/1 -> Add/2, Index Vector/1
  Data/1 -> Index Vector/2
  Index Vector/1 -> SCI Transmit/1
  Add/1 -> While Iterator/1
  Iteration/1 -> Add/1

== system FOC_fieldWeakening/Current Control/SCI_Tx/Code Generation/While Iterator Subsystem1 ==
  Data : Inport
  Iteration : Inport  Port=2
  Add : Sum  Inputs=+-  OutDataTypeStr=Inherit: Same as first input
  Index Vector : MultiPortSwitch  Inputs=1  SaturateOnIntegerOverflow=off  InputSameDT=off
  While Iterator : WhileIterator  MaxIters=-1  WhileBlockType=do-while  ShowIterationPort=on  OutputDataType=int16
  SCI_Data_1 : Outport
  wires:
  While Iterator/1 -> Add/2, Index Vector/1
  Data/1 -> Index Vector/2
  Index Vector/1 -> SCI_Data_1/1
  Add/1 -> While Iterator/1
  Iteration/1 -> Add/1

== system FOC_fieldWeakening/Current Control/SCI_Tx/Code Generation/While Iterator Subsystem2 ==
  Data : Inport
  Iteration : Inport  Port=2
  Add : Sum  Inputs=+-  OutDataTypeStr=Inherit: Same as first input
  Index Vector : MultiPortSwitch  Inputs=1  SaturateOnIntegerOverflow=off  InputSameDT=off
  While Iterator : WhileIterator  MaxIters=-1  WhileBlockType=do-while  ShowIterationPort=on  OutputDataType=int16
  SCI_Data_2 : Outport
  wires:
  While Iterator/1 -> Add/2, Index Vector/1
  Data/1 -> Index Vector/2
  Index Vector/1 -> SCI_Data_2/1
  Add/1 -> While Iterator/1
  Iteration/1 -> Add/1

== system FOC_fieldWeakening/Current Control/SCI_Tx/Code Generation/While Iterator Subsystem3 ==
  Data : Inport
  Iteration : Inport  Port=2
  Add : Sum  Inputs=+-  OutDataTypeStr=Inherit: Same as first input
  Index Vector : MultiPortSwitch  Inputs=1  SaturateOnIntegerOverflow=off  InputSameDT=off
  SCI Transmit : c280xlib/SCI Transmit  sciModule=A  dataHead=''  dataTail=''  frameSize=1  blockingMode=on  outputStatus=off
  While Iterator : WhileIterator  MaxIters=-1  WhileBlockType=do-while  ShowIterationPort=on  OutputDataType=int16
  wires:
  While Iterator/1 -> Add/2, Index Vector/1
  Data/1 -> Index Vector/2
  Index Vector/1 -> SCI Transmit/1
  Add/1 -> While Iterator/1
  Iteration/1 -> Add/1
